simulink model "HydroPower"  (R2024b)
settings: Solver=ode4  StartTime=0.0  StopTime=200  FixedStep=0.001  RelTol=1e-3
values from neighbouring files (symbols this model uses):
  Af = 0.01    [Data__MOTOR.m]    (also in Generator_Data.m = 0.0001; Generator_Datatest.m)
  Bf = 0.0002    [Data__MOTOR.m]    (also in Generator_Data.m = 2e-05; Generator_Datatest.m)
  Cr = 0    [Generator_Data.m]
  CurrentFaultSwitch = 0    [Data__MOTOR.m]    (also in Generator_Data.m = 1; Generator_Datatest.m)
  f = 0.001    [Data__MOTOR.m]    (also in Generator_Data.m = 0)
  J = 0.0012    [Data__MOTOR.m]    (also in Generator_Data.m = 0.263; Generator_Datatest.m = 0.263)
  Ld = 1.4e-3+L_charge    (= 0.0014)    [Generator_Data.m]    (also in Generator_Datatest.m = 0.0231)
  Lq = 2.8e-3+L_charge    (= 0.0028)    [Generator_Data.m]    (also in Generator_Datatest.m = 0.0231)
  P = 4    [Generator_Data.m]    (also in Generator_Datatest.m = 3)
  Phif = 0.8    [Generator_Data.m]
  rate_noise_i = 0.02*In    (= 0.22)    [Data__MOTOR.m]    (also in Generator_Data.m = 0.02; Generator_Datatest.m)
  rate_noise_w = 0.02*Wn    (= 2.96)    [Data__MOTOR.m]    (also in Generator_Data.m = 0.002; Generator_Datatest.m)
  Rs = 0.6+R_charge    (= 0.6)    [Generator_Data.m]    (also in Generator_Datatest.m = 0.48)
  StartStop = 0    [Data__MOTOR.m]    (also in Generator_Data.m; Generator_Datatest.m)
  Te = 0.1    [Data__MOTOR.m]    (also in Generator_Data.m = 1; Generator_Datatest.m)
  Vd = 0    [Generator_Data.m]
  VelocityFaultSwitch = 0    [Data__MOTOR.m]    (also in Generator_Data.m = 1; Generator_Datatest.m)
  Vq = 0    [Generator_Data.m]
  wm = 2*pi*50/P    (= 78.5398163397)    [Generator_Data.m]
undefined symbols (not defined in the file or in its folder): dspblkCoreblockFVToolHelper, gcbh
libraries: SignalEditorBlockLib x3
(part 2 of 3)

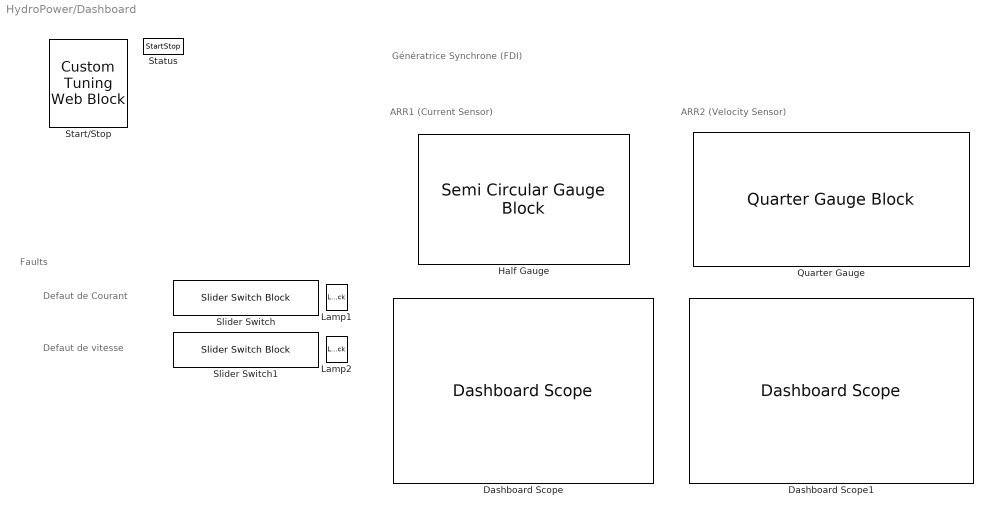
== system HydroPower/Dashboard ==
  note: Faults
  note: ARR2 (Velocity Sensor)
  note: ARR1 (Current Sensor)
  note: Defaut de Courant
  note: Defaut de vitesse
  note: Génératrice Synchrone (FDI)
  Dashboard Scope : DashboardScope  TimeSpan=10000  Ymin=-20  Ymax=20  LegendPosition=Hide  ScaleAtStop=off
  Dashboard Scope1 : DashboardScope  TimeSpan=10000  Ymin=-200  Ymax=200  LegendPosition=Hide  ScaleAtStop=off
  Half Gauge : SemiCircularGaugeBlock  LabelPosition=Hide  ScaleMin=-30  ScaleMax=30
  Lamp1 : LampBlock  LabelPosition=Hide
  Lamp2 : LampBlock  LabelPosition=Hide
  Quarter Gauge : QuarterGaugeBlock  LabelPosition=Hide  ScaleMin=-10  ScaleMax=120
  Slider Switch : SliderSwitchBlock  LabelPosition=Hide
      settings: Values={{'NORMAL', 'FAIL'}, [1 0]}
  Slider Switch1 : SliderSwitchBlock  LabelPosition=Hide
      settings: Values={{'NORMAL', 'FAIL'}, [1 0]}
  Start/Stop : CustomTuningWebBlock  LabelPosition=Hide  ShowInitialText=on  Configuration="{\"components\":[{\"name\":\"BackgroundImageComponent\",\"settings\":{\"image\":{\"size\":[0,0],\"src\":\"default\",\"srcOrientation\":\"Right\"},\"position\":[0,0,1,1],\"scaleMode\":\"0\"}},{\"name\":\"ButtonStateComponent\",\"settings\":{\"buttonType\":\"latch\",\"clickFcn\":\"if(StartStop==0)\\n    StartStop=1;\\n\\n\\n    set_param('DC_moteor_fdi1', 'SimulationCommand', 'start');\\n\\nelse\\n    StartStop=0;\\n\\n\\n    set_param('DC_moteor_fdi1', 'SimulationCommand', 'stop');\\n\\nend\",\"image\":{\"size\":[180,45],\"srcOrientation\":\"Right\"},\"latched\":false,\"offValue\":null,\"onValue\":\"1\",\"position\":[0,0,1,1],\"pressDelay\":\"500\",\"pressFcn\":\"\",\"repeatInterval\":\"0\",\"states\":[{\"horizontalAlignment\":\"center\",\"image\":{\"position\":[0.016452872281093156,0,1,0.9670942554378137],\"size\":[1,0.9670942554378137],\"src\":\"data:image\\/jpeg;base64,\\/9j\\/4AAQSkZJRgABAQEASABIAAD\\/4QKyRXhpZgAATU0AKgAAAAgAAodpAAQAAAABAAABMuocAAcAAAEMAAAAJgAAAAAc6gAAAAEAAAAAAAAAAAAAAAAAAAAAAAAAAAAAAAAAAAAAAAAAAAAAAAAAAAAAAAAAAAAAAAAAAAAAAAAAAAAAAAAAAAAAAAAAAAAAAAAAAAAAAAAAAAAAAAAAAAAAAAAAAAAAAAAAAAAAAAAAAAAAAAAAAAAAAAAAAAAAAAAAAAAAAAAAAAAAAAAAAAAAAAAAAAAAAAAAAAAAAAAAAAAAAAAAAAAAAAAAAAAAAAAAAAAAAAAAAAAAAAAAAAAAAAAAAAAAAAAAAAAAAAAAAAAAAAAAAAAAAAAAAAAAAAAAAAAAAA ...(+45438 chars)\",\"srcOrientation\":\"Right\"},\"label\":{\"color\":[1,1,0.78,1],\"icon\":{\"size\":[0,0],\"src\":\"default\",\"srcOrientation\":\"Right\"},\"iconOffset\":0,\"iconPlacement\":\"left\",\"opacity\":1,\"show\":true,\"text\":{\"content\":\"\",\"font\":\"Helvetica\"}},\"labelOffset\":[0,0],\"verticalAlignment\":\"middle\"},{\"horizontalAlignment\":\"center\",\"image\":{\"position\":[0.015461997019374063,0,1,0.9690760059612519],\"size\":[1,0.9690760059612519],\"src\":\"data:image\\/jpeg;base64,\\/9j\\/4AAQSkZJRgABAQEASABIAAD\\/4QKyRXhpZgAATU0AKgAAAAgAAodpAAQAAAABAAABMuocAAcAAAEMAAAAJgAAAAAc6gAAAAEAAAAAAAAAAAAAAAAAAAAAAAAAAAAAAAAAAAAAAAAAAAAAAAAAAAAAAAAAAAAAAAAAAAAAAAAAAAAAAAAAAAAAAAAAAAAAAAAAAAAAAAAAAAAAAAAAAAAAAAAAAAAAAAAAAAAAAAAAAAAAAAAAAAAAAAAAAAAAAAAAAAAAAAAAAAAAAAAAAAAAAAAAAAAAAAAAAAAAAAAAAAAAAAAAAAAAAAAAAAAAAAAAAAAAAAAAAAAAAAAAAAAAAAAAAAAAAAAAAAAAAAAAAAAAAAAAAAAAAAAAAAAAAAAAAAAAAA ...(+48838 chars)\",\"srcOrientation\":\"Right\"},\"label\":{\"color\":[1,1,0.78,1],\"icon\":{\"size\":[0,0],\"src\":\"default\",\"srcOrientation\":\"Right\"},\"iconOffset\":0,\"iconPlacement\":\"left\",\"opacity\":1,\"show\":true,\"text\":{\"content\":\"\",\"font\":\"Helvetica\"}},\"labelOffset\":[0,0],\"verticalAlignment\":\"middle\"},{\"horizontalAlignment\":\"center\",\"image\":{\"position\":[0.015461997019374063,0,1,0.9690760059612519],\"size\":[1,0.9690760059612519],\"src\":\"data:image\\/jpeg;base64,\\/9j\\/4AAQSkZJRgABAQEASABIAAD\\/4QKyRXhpZgAATU0AKgAAAAgAAodpAAQAAAABAAABMuocAAcAAAEMAAAAJgAAAAAc6gAAAAEAAAAAAAAAAAAAAAAAAAAAAAAAAAAAAAAAAAAAAAAAAAAAAAAAAAAAAAAAAAAAAAAAAAAAAAAAAAAAAAAAAAAAAAAAAAAAAAAAAAAAAAAAAAAAAAAAAAAAAAAAAAAAAAAAAAAAAAAAAAAAAAAAAAAAAAAAAAAAAAAAAAAAAAAAAAAAAAAAAAAAAAAAAAAAAAAAAAAAAAAAAAAAAAAAAAAAAAAAAAAAAAAAAAAAAAAAAAAAAAAAAAAAAAAAAAAAAAAAAAAAAAAAAAAAAAAAAAAAAAAAAAAAAAAAAAAAAA ...(+48838 chars)\",\"srcOrientation\":\"Right\"},\"label\":{\"color\":[1,1,0.78,1],\"icon\":{\"size\":[0,0],\"src\":\"default\",\"srcOrientation\":\"Right\"},\"iconOffset\":0,\"iconPlacement\":\"left\",\"opacity\":1,\"show\":true,\"text\":{\"content\":\"\",\"font\":\"Helvetica\"}},\"labelOffset\":[0,0],\"verticalAlignment\":\"middle\"},{\"horizontalAlignment\":\"center\",\"image\":{\"position\":[0.015461997019374063,0,1,0.9690760059612519],\"size\":[1,0.9690760059612519],\"src\":\"data:image\\/jpeg;base64,\\/9j\\/4AAQSkZJRgABAQEASABIAAD\\/4QKyRXhpZgAATU0AKgAAAAgAAodpAAQAAAABAAABMuocAAcAAAEMAAAAJgAAAAAc6gAAAAEAAAAAAAAAAAAAAAAAAAAAAAAAAAAAAAAAAAAAAAAAAAAAAAAAAAAAAAAAAAAAAAAAAAAAAAAAAAAAAAAAAAAAAAAAAAAAAAAAAAAAAAAAAAAAAAAAAAAAAAAAAAAAAAAAAAAAAAAAAAAAAAAAAAAAAAAAAAAAAAAAAAAAAAAAAAAAAAAAAAAAAAAAAAAAAAAAAAAAAAAAAAAAAAAAAAAAAAAAAAAAAAAAAAAAAAAAAAAAAAAAAAAAAAAAAAAAAAAAAAAAAAAAAAAAAAAAAAAAAAAAAAAAAAAAAAAAAA ...(+48838 chars)\",\"srcOrientation\":\"Right\"},\"label\":{\"color\":[1,1,0.78,1],\"icon\":{\"size\":[0,0],\"src\":\"default\",\"srcOrientation\":\"Right\"},\"iconOffset\":0,\"iconPlacement\":\"left\",\"opacity\":1,\"show\":true,\"text\":{\"content\":\"\",\"font\":\"Helvetica\"}},\"labelOffset\":[0,0],\"verticalAlignment\":\"middle\"}]}},{\"name\":\"ForegroundImageComponent\",\"settings\":{\"image\":{\"size\":[0,0],\"src\":\"default\",\"srcOrientation\":\"horizontal\"},\"isForeground\":1,\"position\":[0,0,1,1],\"scaleMode\":\"0\"}}],\"settings\":{\"BindingType\":\"param\",\"aspectRatio\":3.7777777777777777,\"backgroundColor\":[0,0,0,\"1\"],\"backgroundOffset\":0,\"backgroundOpacity\":1,\"fixedAspectRatio\":\"off\",\"foregroundColor\":[252,252,196],\"showBackgroundColor\":false,\"variant\":\"push\",\"version\":\"R2024b\"},\"type\":\"Button\"}"
  Status : Constant  Value=StartStop
